simulink library "lib_Convection_HexagonRodCrossFlowHilpert"  (R2015a)
settings: Solver=ode45  StartTime=0.0  StopTime=10.0  RelTol=1e-3
libraries: simulink x12, lib_GenTools_MinMax x1
settings Model: Creator=jlkratz  LastModifiedBy=jlkratz

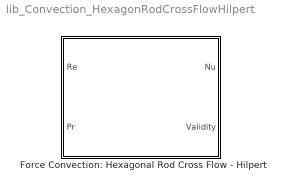
== system lib_Convection_HexagonRodCrossFlowHilpert ==
  Force Convection: Hexagonal Rod Cross Flow - Hilpert : Subsystem  mask(TSAT: Hexagonal Rod Cross Flow - Hilpert){PointOrFace_M=Flow directed at a point of the hexagon}
      mask help:
      | This block estimates the average Nusselt number of an external flow over an isothermal rod with a hexagonal cross-section. The correlation employed was originally developed by Hilpert and has been modified to address non-circular cross-sectional shapes. It has options to address the case in which the flow is directed at a point of the hexagon or a side. Note that when the flow is directed at a face, the Reynolds number should be calculated based on the length from opposite sides of the hexagon and when the flow is directed at a point, the Reynolds number should be calculated based on the length from opposite points of the hexagon. The properties of the fluid should be evaluated at the film temperature. The correlation is subject to the following restrictions:
      |
      | Flow directed at a point of the hexagon:
      | 4500 <= Re <= 90700
      | Pr >= 0.7
      |
      | Flow directed at a side of the hexagon:
      | 5200 <= Re <= 105000
      | Pr >= 0.7
      |
      | Re is the Reynolds number and Pr is the Prandtl number. For more information see the block help menu.
      mask Help: web(which('Convection_TSAT_HexagonRodCrossFlowHilpert.html'),'-helpbrowser')
      mask TypeOptions PointOrFace_M: Flow directed at a point of the hexagon | Flow directed at a side of the hexagon

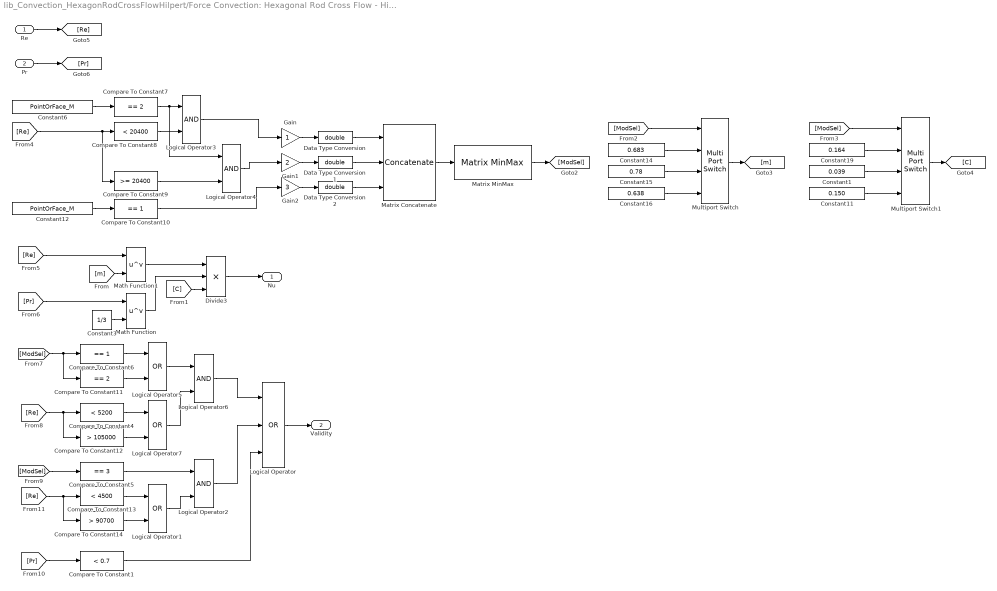
== system lib_Convection_HexagonRodCrossFlowHilpert/Force Convection: Hexagonal Rod Cross Flow - Hilpert ==
  Re : Inport
  Pr : Inport  Port=2
  Compare To Constant1 : simulink/Logic and Bit Operations/Compare To Constant  relop=<  const=0.7  OutDataTypeStr=boolean
  Compare To Constant10 : simulink/Logic and Bit Operations/Compare To Constant  relop===  const=1  OutDataTypeStr=boolean
  Compare To Constant11 : simulink/Logic and Bit Operations/Compare To Constant  relop===  const=2  OutDataTypeStr=boolean
  Compare To Constant12 : simulink/Logic and Bit Operations/Compare To Constant  relop=>  const=105000  OutDataTypeStr=boolean
  Compare To Constant13 : simulink/Logic and Bit Operations/Compare To Constant  relop=<  const=4500  OutDataTypeStr=boolean
  Compare To Constant14 : simulink/Logic and Bit Operations/Compare To Constant  relop=>  const=90700  OutDataTypeStr=boolean
  Compare To Constant4 : simulink/Logic and Bit Operations/Compare To Constant  relop=<  const=5200  OutDataTypeStr=boolean
  Compare To Constant5 : simulink/Logic and Bit Operations/Compare To Constant  relop===  const=3  OutDataTypeStr=boolean
  Compare To Constant6 : simulink/Logic and Bit Operations/Compare To Constant  relop===  const=1  OutDataTypeStr=boolean
  Compare To Constant7 : simulink/Logic and Bit Operations/Compare To Constant  relop===  const=2  OutDataTypeStr=boolean
  Compare To Constant8 : simulink/Logic and Bit Operations/Compare To Constant  relop=<  const=20400  OutDataTypeStr=boolean
  Compare To Constant9 : simulink/Logic and Bit Operations/Compare To Constant  relop=>=  const=20400  OutDataTypeStr=boolean
  Constant1 : Constant  Value=0.039
  Constant11 : Constant  Value=0.150
  Constant12 : Constant  Value=PointOrFace_M
  Constant14 : Constant  Value=0.683
  Constant15 : Constant  Value=0.78
  Constant16 : Constant  Value=0.638
  Constant19 : Constant  Value=0.164
  Constant3 : Constant  Value=1/3
  Constant6 : Constant  Value=PointOrFace_M
  Data Type Conversion : DataTypeConversion  OutDataTypeStr=double
  Data Type Conversion1 : DataTypeConversion  OutDataTypeStr=double
  Data Type Conversion2 : DataTypeConversion  OutDataTypeStr=double
  Divide3 : Product  Inputs=***
  Gain : Gain
  Gain1 : Gain  Gain=2
  Gain2 : Gain  Gain=3
  Logical Operator : Logic  Operator=OR  Inputs=3  AllPortsSameDT=off  OutDataTypeStr=boolean
  Logical Operator1 : Logic  Operator=OR  AllPortsSameDT=off  OutDataTypeStr=boolean
  Logical Operator{2..4,6} (4 alike) : Logic  AllPortsSameDT=off  OutDataTypeStr=boolean
  Logical Operator5 : Logic  Operator=OR  AllPortsSameDT=off  OutDataTypeStr=boolean
  Logical Operator7 : Logic  Operator=OR  AllPortsSameDT=off  OutDataTypeStr=boolean
  Math Function : Math  Operator=pow  SaturateOnIntegerOverflow=on
  Math Function1 : Math  Operator=pow  SaturateOnIntegerOverflow=on
  Matrix Concatenate : Concatenate  NumInputs=3  Mode=Multidimensional array  ConcatenateDimension=2
  Matrix MinMax : lib_GenTools_MinMax/Matrix MinMax  rows_M=on  cols_M=off  all_M=off  minmax_M=off  BN_M=gcb
  Multiport Switch : MultiPortSwitch
  Multiport Switch1 : MultiPortSwitch
  Nu : Outport
  Validity : Outport  Port=2
  wires:
  Compare To Constant1/1 -> Logical Operator/3
  [Pr] -> Compare To Constant1/1
  Logical Operator2/1 -> Logical Operator/2
  Logical Operator6/1 -> Logical Operator/1
  Compare To Constant5/1 -> Logical Operator2/1
  Logical Operator1/1 -> Logical Operator2/2
  Compare To Constant14/1 -> Logical Operator1/2
  Compare To Constant13/1 -> Logical Operator1/1
  [Re] -> Compare To Constant14/1, Compare To Constant13/1
  [ModSel] -> Compare To Constant5/1
  Logical Operator5/1 -> Logical Operator6/1
  Logical Operator7/1 -> Logical Operator6/2
  Compare To Constant12/1 -> Logical Operator7/2
  Compare To Constant4/1 -> Logical Operator7/1
  [Re] -> Compare To Constant4/1, Compare To Constant12/1
  Compare To Constant11/1 -> Logical Operator5/2
  Compare To Constant6/1 -> Logical Operator5/1
  [ModSel] -> Compare To Constant6/1, Compare To Constant11/1
  Pr/1 -> [Pr]
  Re/1 -> [Re]
  [Pr] -> Math Function/1
  [Re] -> Math Function1/1
  Constant12/1 -> Compare To Constant10/1
  Compare To Constant9/1 -> Logical Operator4/2
  Compare To Constant8/1 -> Logical Operator3/2
  Compare To Constant7/1 -> Logical Operator3/1, Logical Operator4/1
  [Re] -> Compare To Constant8/1, Compare To Constant9/1
  Constant6/1 -> Compare To Constant7/1
  Matrix Concatenate/1 -> Matrix MinMax/1
  Data Type Conversion2/1 -> Matrix Concatenate/3
  Data Type Conversion1/1 -> Matrix Concatenate/2
  Data Type Conversion/1 -> Matrix Concatenate/1
  Matrix MinMax/1 -> [ModSel]
  Constant11/1 -> Multiport Switch1/4
  Constant1/1 -> Multiport Switch1/3
  Constant19/1 -> Multiport Switch1/2
  Constant16/1 -> Multiport Switch/4
  Constant15/1 -> Multiport Switch/3
  Constant14/1 -> Multiport Switch/2
  Multiport Switch1/1 -> [C]
  Multiport Switch/1 -> [m]
  [ModSel] -> Multiport Switch1/1
  [ModSel] -> Multiport Switch/1
  Logical Operator3/1 -> Gain/1
  Logical Operator4/1 -> Gain1/1
  Compare To Constant10/1 -> Gain2/1
  Gain2/1 -> Data Type Conversion2/1
  Gain1/1 -> Data Type Conversion1/1
  Gain/1 -> Data Type Conversion/1
  Logical Operator/1 -> Validity/1
  [C] -> Divide3/3
  Divide3/1 -> Nu/1
  Math Function1/1 -> Divide3/1
  [m] -> Math Function1/2
  Constant3/1 -> Math Function/2
  Math Function/1 -> Divide3/2
